simulink model "UIO_example_EEG_2ch_discrete"  (R2019b)
settings: Solver=FixedStepAuto  StartTime=0.0  StopTime=60  FixedStep=dt  RelTol=1e-3
values from neighbouring files (symbols this model uses):
  B2 = [68245 0 0;0 -2 0;0 0 2;0 232.75 0; 0 0 -232.75]    [UIO_adaptive_example.m]    (also in UIO_adaptive_example_2.m = [1;0;1;0]; UIO_adaptive_example_EEG.m = ones(opt_order,1); UIO_adaptive_example_EEG_Balas_2ch.m = ones(opt_order,1); UIO_adaptive_example_EEG_ch2.m = ones(opt_order,1))
  F = B2'*P/(C)    [UIO_adaptive_example_2.m]    (also in UIO_adaptive_example_EEG.m = B2'*P/(C_data{opt_order}); UIO_adaptive_example_EEG_ch2.m = B2'*P/(C_data{opt_order}); UIO_adaptive_example_EEG_ch2_DEAP.m = B2'*P/(C_data{opt_order}); UIO_adaptive_example_EEG_ch2_ECEO.m = B2'*P/(C_data{opt_order}))
  Gamma = 20    [UIO_adaptive_example_2.m]    (also in UIO_adaptive_example_EEG.m = 0.001; UIO_adaptive_example_EEG_ch2.m = loop(i); UIO_adaptive_example_EEG_ch2_DEAP.m = loop(i); UIO_adaptive_example_EEG_ch2_ECEO.m = loop(i))
  L = inv(P)*Y    [UIO_adaptive_example.m]    (also in UIO_adaptive_example_2.m; UIO_adaptive_example_EEG.m; UIO_adaptive_example_EEG_ch2.m; UIO_adaptive_example_EEG_ch2_DEAP.m)
  opt_order = 20    [UIO_adaptive_example_EEG.m]    (also in UIO_adaptive_example_EEG_Balas_2ch.m = 4; UIO_adaptive_example_EEG_ch2.m = 4; UIO_adaptive_example_EEG_ch2_DEAP.m = 4; UIO_adaptive_example_EEG_ch2_ECEO.m = 4)
undefined symbols (not defined in the file or in its folder): sigbuilder_block
settings Model: Creator=Tris  LastModifiedBy=Tris
settings DataIOCC: ExternalInput=Y_sim1, Y_sim2  LoadExternalInput=on

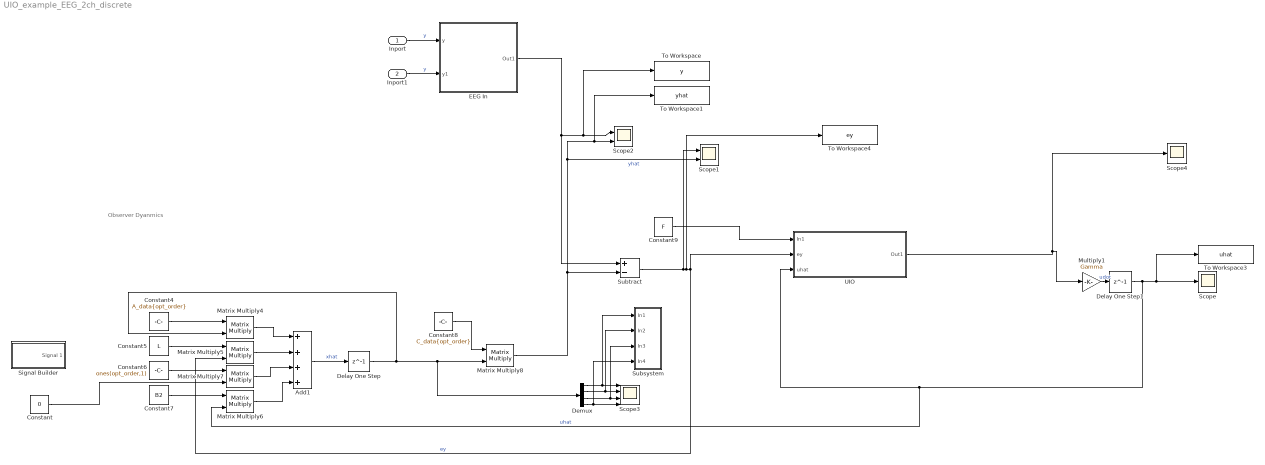
== system UIO_example_EEG_2ch_discrete ==
  note: Observer Dyanmics
  Inport : Inport
  Inport1 : Inport  Port=2
  Add1 : Sum  Inputs=++++
  Constant : Constant  Value=0
  Constant4 : Constant  Value=A_data{opt_order}  VectorParams1D=off
  Constant5 : Constant  Value=L  VectorParams1D=off
  Constant6 : Constant  Value=ones(opt_order,1)  VectorParams1D=off
  Constant7 : Constant  Value=B2  VectorParams1D=off
  Constant8 : Constant  Value=C_data{opt_order}  VectorParams1D=off
  Constant9 : Constant  Value=F  VectorParams1D=off
  Delay One Step : Delay  DelayLength=1
  Delay One Step1 : Delay  DelayLength=1
  Demux : Demux
  EEG In : Subsystem
  Matrix Multiply{4..8} (5 alike) : Product  Multiplication=Matrix(*)
  Multiply1 : Gain  Gain=Gamma
  Scope : Scope
  Scope1 : Scope  NumInputPorts=2
  Scope2 : Scope  NumInputPorts=2
  Scope3 : Scope  NumInputPorts=4
  Scope4 : Scope
  Signal Builder : Subsystem  Tag=STV Subsys  LoadFcn=sigbuilder_block('load');  StartFcn=sigbuilder_block('start');  StopFcn=sigbuilder_block('stop');  ClipboardFcn=sigbuilder_block('clipboard');  mask(Sigbuilder block){tuvar=[0:10]}
      mask help: Simulink:masks:SigbuilderBlock_MD
      mask init:
      | if ~strcmp(get_param(bdroot(gcbh),'SimulationStatus'),'stopped') tuvar = sigbuilder_block('maskInit'); end
      settings: CopyFcn=sigbuilder_block('copy');  DeleteFcn=sigbuilder_block('delete');  ModelCloseFcn=sigbuilder_block('modelClose');  PreSaveFcn=sigbuilder_block('preSave');  PauseFcn=sigbuilder_block('pause');  ContinueFcn=sigbuilder_block('continue');  NameChangeFcn=sigbuilder_block('namechange');  OpenFcn=sigbuilder_block('open',[437.6 199.2 550.4 400 ]);  CloseFcn=sigbuilder_block('close');
      mask Display: plot(0, 0, 100, 100,[2, 2, 32, 32, 2], [68, 8, 8, 68, 68],[32, 2], [38, 38], [32, 19, 2],[53, 60, 44], [32, 17, 17, 2],[16, 16, 31, 31]);txt = getActiveGroup(gcbh);text(2, 100, txt,'verticalAlignment', 'top');
  Subsystem : Subsystem
  Subtract : Sum  Inputs=+-
  To Workspace : ToWorkspace  VariableName=y  SaveFormat=Timeseries  SampleTime=-1
  To Workspace1 : ToWorkspace  VariableName=yhat  SaveFormat=Timeseries  SampleTime=-1
  To Workspace3 : ToWorkspace  VariableName=uhat  SaveFormat=Timeseries  SampleTime=-1
  To Workspace4 : ToWorkspace  VariableName=ey  SaveFormat=Timeseries  SampleTime=-1
  UIO : Subsystem
  wires:
  Matrix Multiply5/1 -> Add1/2
  Matrix Multiply4/1 -> Add1/1
  Matrix Multiply7/1 -> Add1/3
  Matrix Multiply6/1 -> Add1/4
  Constant4/1 -> Matrix Multiply4/1
  Constant5/1 -> Matrix Multiply5/1
  Constant6/1 -> Matrix Multiply7/1
  Add1/1 -> Delay One Step/1  "xhat"
  Matrix Multiply8/1 -> To Workspace1/1, Scope2/2, Scope1/2, Subtract/2  "yhat"
  Subtract/1 -> To Workspace4/1, Matrix Multiply5/2, UIO/2(ey), Scope1/1  "ey"
  Delay One Step1/1 -> To Workspace3/1, Scope/1, UIO/3(uhat), Matrix Multiply6/2  "uhat"
  Constant8/1 -> Matrix Multiply8/1
  Multiply1/1 -> Delay One Step1/1  "udot"
  Demux/1 -> Subsystem/1(In1), Scope3/1
  Demux/2 -> Subsystem/2(In2), Scope3/2
  Demux/3 -> Subsystem/3(In3), Scope3/3
  Demux/4 -> Subsystem/4(In4), Scope3/4
  Constant7/1 -> Matrix Multiply6/1
  Constant/1 -> Matrix Multiply7/2
  Delay One Step/1 -> Demux/1, Matrix Multiply8/2, Matrix Multiply4/2
  UIO/1(Out1) -> Scope4/1, Multiply1/1
  Constant9/1 -> UIO/1(In1)
  EEG In/1(Out1) -> Subtract/1, To Workspace/1, Scope2/1
  Inport/1 -> EEG In/1(y)  "y"
  Inport1/1 -> EEG In/2(y1)  "y"

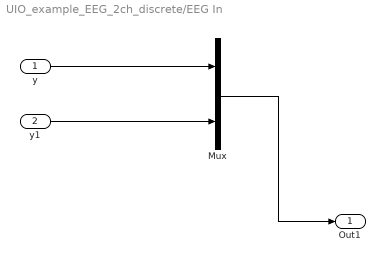
== system UIO_example_EEG_2ch_discrete/EEG In ==
  y : Inport
  y1 : Inport  Port=2
  Mux : Mux  Inputs=2
  Out1 : Outport
  wires:
  y1/1 -> Mux/2
  y/1 -> Mux/1
  Mux/1 -> Out1/1

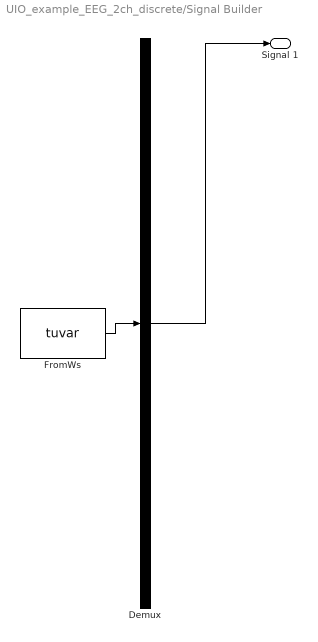
== system UIO_example_EEG_2ch_discrete/Signal Builder ==
  Demux : Demux  Tag=STV Demux  Outputs=1
  FromWs : FromWorkspace  Tag=STV FromWs  VariableName=tuvar  SampleTime=0
      SigBuilderData=|
      | common.afterFinalStr = 'Extrapolate'
      | common.sampleTime = 0
      | dataSet.timeRange = [0 60]
      | dataSet.name = 'Group 1'
      | sbobj.Groups.Name = 'Group 1'
      | sbobj.Groups.Signals.Name = 'Signal 1'
      | sbobj.Groups.Signals.XData = [0 18 18 19 19 60]
      | sbobj.Groups.Signals.YData = [0 0 1 1 0 0]
      | sbobj.Groups.TimeRange = [0 60]
  Signal 1 : Outport  Tag=STV Outport
  wires:
  Demux/1 -> Signal 1/1
  FromWs/1 -> Demux/1

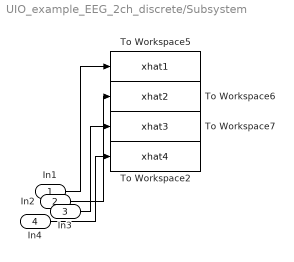
== system UIO_example_EEG_2ch_discrete/Subsystem ==
  In1 : Inport
  In2 : Inport  Port=2
  In3 : Inport  Port=3
  In4 : Inport  Port=4
  To Workspace2 : ToWorkspace  VariableName=xhat4  SaveFormat=Timeseries  SampleTime=-1
  To Workspace5 : ToWorkspace  VariableName=xhat1  SaveFormat=Timeseries  SampleTime=-1
  To Workspace6 : ToWorkspace  VariableName=xhat2  SaveFormat=Timeseries  SampleTime=-1
  To Workspace7 : ToWorkspace  VariableName=xhat3  SaveFormat=Timeseries  SampleTime=-1
  wires:
  In1/1 -> To Workspace5/1
  In4/1 -> To Workspace2/1
  In2/1 -> To Workspace6/1
  In3/1 -> To Workspace7/1

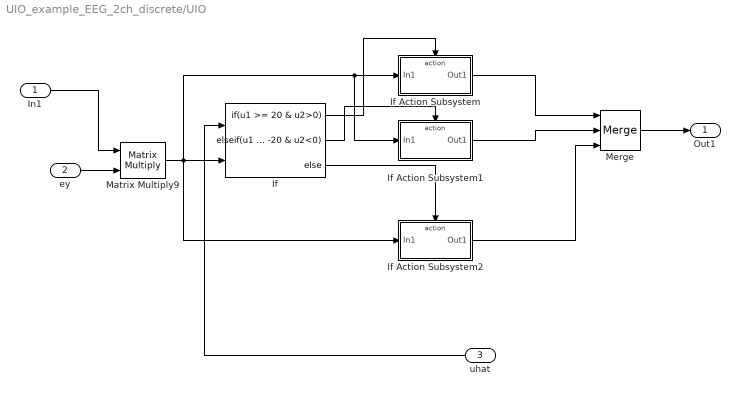
== system UIO_example_EEG_2ch_discrete/UIO ==
  In1 : Inport
  ey : Inport  Port=2
  uhat : Inport  Port=3
  If : If  NumInputs=2  IfExpression=u1 >= 20 & u2>0  ElseIfExpressions=u1 <= -20 & u2<0
  If Action Subsystem : Subsystem  TreatAsAtomicUnit=on
  If Action Subsystem1 : Subsystem  TreatAsAtomicUnit=on
  If Action Subsystem2 : Subsystem  TreatAsAtomicUnit=on
  Matrix Multiply9 : Product  Multiplication=Matrix(*)
  Merge : Merge  Inputs=3
  Out1 : Outport
  wires:
  If/2 -> If Action Subsystem1/Action
  If/3 -> If Action Subsystem2/Action
  Matrix Multiply9/1 -> If/2, If Action Subsystem2/1(In1), If Action Subsystem1/1(In1), If Action Subsystem/1(In1)
  If Action Subsystem2/1(Out1) -> Merge/3
  If Action Subsystem/1(Out1) -> Merge/1
  If Action Subsystem1/1(Out1) -> Merge/2
  ey/1 -> Matrix Multiply9/2
  If/1 -> If Action Subsystem/Action
  uhat/1 -> If/1
  In1/1 -> Matrix Multiply9/1
  Merge/1 -> Out1/1

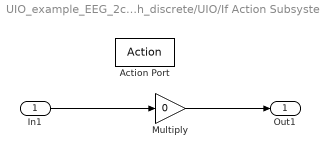
== system UIO_example_EEG_2ch_discrete/UIO/If Action Subsystem ==
  In1 : Inport
  Action Port : ActionPort  ActionPortLabel=if(u1 >= 20 & u2>0)
  Multiply : Gain  Gain=0
  Out1 : Outport
  wires:
  In1/1 -> Multiply/1
  Multiply/1 -> Out1/1

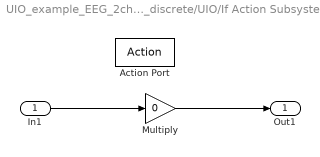
== system UIO_example_EEG_2ch_discrete/UIO/If Action Subsystem1 ==
  In1 : Inport
  Action Port : ActionPort  ActionPortLabel=elseif(u1 <= -20 & u2<0)
  Multiply : Gain  Gain=0
  Out1 : Outport
  wires:
  In1/1 -> Multiply/1
  Multiply/1 -> Out1/1

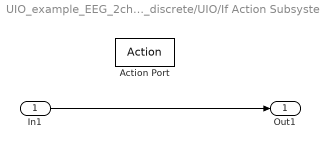
== system UIO_example_EEG_2ch_discrete/UIO/If Action Subsystem2 ==
  In1 : Inport
  Action Port : ActionPort  ActionPortLabel=else
  Out1 : Outport
  wires:
  In1/1 -> Out1/1
